simulink model "Lateral_Dynamics_2Track"  (R2020a)
settings: Solver=VariableStepAuto  StartTime=0.0  StopTime=10.0  RelTol=1e-3
values from neighbouring files (symbols this model uses):
  Brake_radius = 0.1    [Properties.sldd]
  Car_mass = 245.0    [Properties.sldd]
  CG_x = 0.6    [Properties.sldd]
  Effective_radius = 0.2    [Properties.sldd]
  Track_width = 2.0    [Properties.sldd]
  Wheel_inertia = 0.0205    [Properties.sldd]
  Wheelbase = 1.2    [Properties.sldd]
undefined symbols (not defined in the file or in its folder): Car_Iz
libraries: simulink x2
settings Model: Creator=Matthew  LastModifiedBy=Matthew

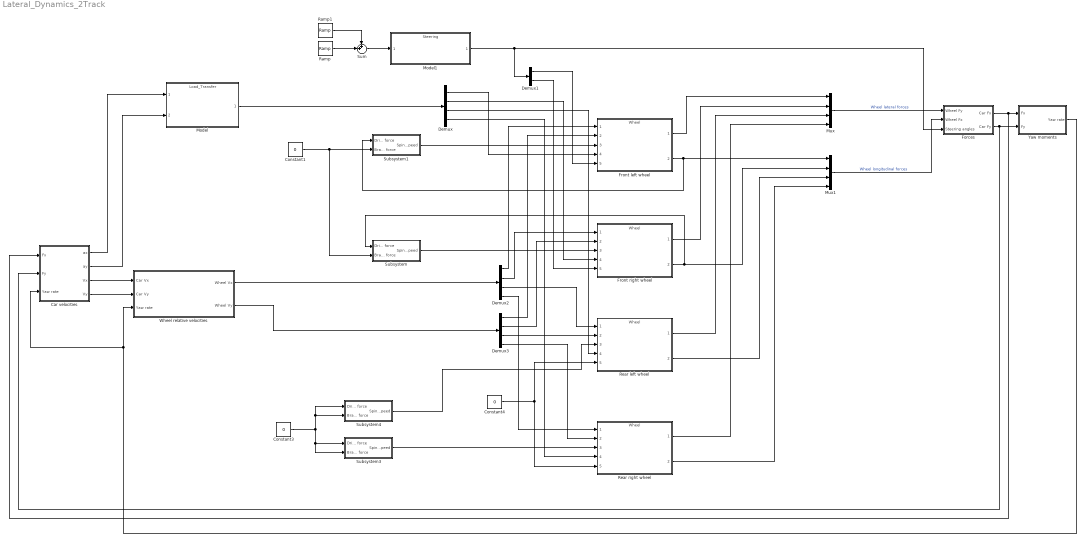
== system Lateral_Dynamics_2Track ==
  Car velocities : Subsystem
  Constant1 : Constant  Value=0
  Constant3 : Constant  Value=0
  Constant4 : Constant  Value=0
  Demux : Demux
  Demux1 : Demux  Outputs=2
  Demux2 : Demux
  Demux3 : Demux
  Forces : Subsystem
  Front left wheel : ModelReference  ModelNameDialog=Wheel  SimulationMode=Normal  ModelReferenceVersion=1.8
  Front right wheel : ModelReference  ModelNameDialog=Wheel  SimulationMode=Normal  ModelReferenceVersion=1.8
  Model : ModelReference  ModelNameDialog=Load_Transfer  SimulationMode=Normal  ModelReferenceVersion=1.23
  Model1 : ModelReference  ModelNameDialog=Steering  SimulationMode=Normal  ModelReferenceVersion=1.2
  Mux : Mux
  Mux1 : Mux
  Ramp : simulink/Sources/Ramp  slope=0.05  start=0  InitialOutput=0
  Ramp1 : simulink/Sources/Ramp  slope=-0.05  start=2  InitialOutput=0
  Rear left wheel : ModelReference  ModelNameDialog=Wheel  SimulationMode=Normal  ModelReferenceVersion=1.8
  Rear right wheel : ModelReference  ModelNameDialog=Wheel  SimulationMode=Normal  ModelReferenceVersion=1.8
  Subsystem : Subsystem
  Subsystem1 : Subsystem
  Subsystem3 : Subsystem
  Subsystem4 : Subsystem
  Sum : Sum  Inputs=++|
  Wheel relative velocities : Subsystem
  Yaw moments : Subsystem
  wires:
  Subsystem/1(Spin speed) -> Front right wheel/3
  Demux/2 -> Front right wheel/4
  Model/1 -> Demux/1
  Subsystem1/1(Spin speed) -> Front left wheel/3
  Car velocities/1(ax) -> Model/1
  Demux/1 -> Front left wheel/4
  Front left wheel/1 -> Mux/1
  Front right wheel/1 -> Mux/2
  Constant1/1 -> Subsystem/2(Brake force), Subsystem1/2(Brake force)
  Wheel relative velocities/1(Wheel Vx) -> Demux2/1
  Wheel relative velocities/2(Wheel Vy) -> Demux3/1
  Demux2/1 -> Front left wheel/1
  Demux3/1 -> Front left wheel/2
  Demux2/2 -> Front right wheel/1
  Demux3/2 -> Front right wheel/2
  Subsystem4/1(Spin speed) -> Rear left wheel/3
  Constant3/1 -> Subsystem4/2(Brake force), Subsystem4/1(Drive force), Subsystem3/2(Brake force), Subsystem3/1(Drive force)
  Rear left wheel/1 -> Mux/3
  Rear right wheel/1 -> Mux/4
  Front left wheel/2 -> Subsystem1/1(Drive force), Mux1/1
  Front right wheel/2 -> Subsystem/1(Drive force), Mux1/2
  Rear left wheel/2 -> Mux1/3
  Rear right wheel/2 -> Mux1/4
  Mux/1 -> Forces/1(Wheel Fy)  "Wheel lateral forces"
  Mux1/1 -> Forces/2(Wheel Fx)  "Wheel longitudinal forces"
  Model1/1 -> Forces/3(Steering angles), Demux1/1
  Constant4/1 -> Rear left wheel/5, Rear right wheel/5
  Subsystem3/1(Spin speed) -> Rear right wheel/3
  Demux2/3 -> Rear left wheel/1
  Demux2/4 -> Rear right wheel/1
  Demux3/3 -> Rear left wheel/2
  Demux3/4 -> Rear right wheel/2
  Demux1/1 -> Front left wheel/5
  Demux1/2 -> Front right wheel/5
  Forces/1(Car Fx) -> Car velocities/1(Fx), Yaw moments/1(Fx)
  Forces/2(Car Fy) -> Car velocities/2(Fy), Yaw moments/2(Fy)
  Yaw moments/1(Yaw rate) -> Car velocities/3(Yaw rate), Wheel relative velocities/3(Yaw rate)
  Demux/3 -> Rear left wheel/4
  Demux/4 -> Rear right wheel/4
  Car velocities/3(Vx) -> Wheel relative velocities/1(Car Vx)
  Car velocities/4(Vy) -> Wheel relative velocities/2(Car Vy)
  Car velocities/2(ay) -> Model/2
  Sum/1 -> Model1/1
  Ramp1/1 -> Sum/1
  Ramp/1 -> Sum/2

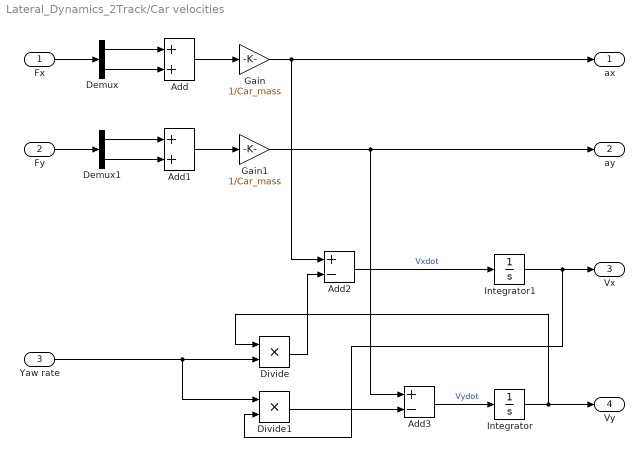
== system Lateral_Dynamics_2Track/Car velocities ==
  Fx : Inport
  Fy : Inport  Port=2
  Yaw rate : Inport  Port=3
  Add : Sum  Inputs=2
  Add1 : Sum  Inputs=2
  Add2 : Sum  Inputs=+-
  Add3 : Sum  Inputs=+-
  Demux : Demux  Outputs=2
  Demux1 : Demux  Outputs=2
  Divide : Product  Inputs=**
  Divide1 : Product  Inputs=**
  Gain : Gain  Gain=1/Car_mass
  Gain1 : Gain  Gain=1/Car_mass
  Integrator : Integrator
  Integrator1 : Integrator
  ax : Outport
  ay : Outport  Port=2
  Vx : Outport  Port=3
  Vy : Outport  Port=4
  wires:
  Fx/1 -> Demux/1
  Demux/1 -> Add/1
  Demux/2 -> Add/2
  Fy/1 -> Demux1/1
  Demux1/1 -> Add1/1
  Demux1/2 -> Add1/2
  Add/1 -> Gain/1
  Add1/1 -> Gain1/1
  Gain/1 -> ax/1, Add2/1
  Gain1/1 -> Add3/1, ay/1
  Integrator1/1 -> Divide1/2, Vx/1
  Integrator/1 -> Vy/1, Divide/1
  Yaw rate/1 -> Divide1/1, Divide/2
  Divide/1 -> Add2/2
  Divide1/1 -> Add3/2
  Add3/1 -> Integrator/1  "Vydot"
  Add2/1 -> Integrator1/1  "Vxdot"

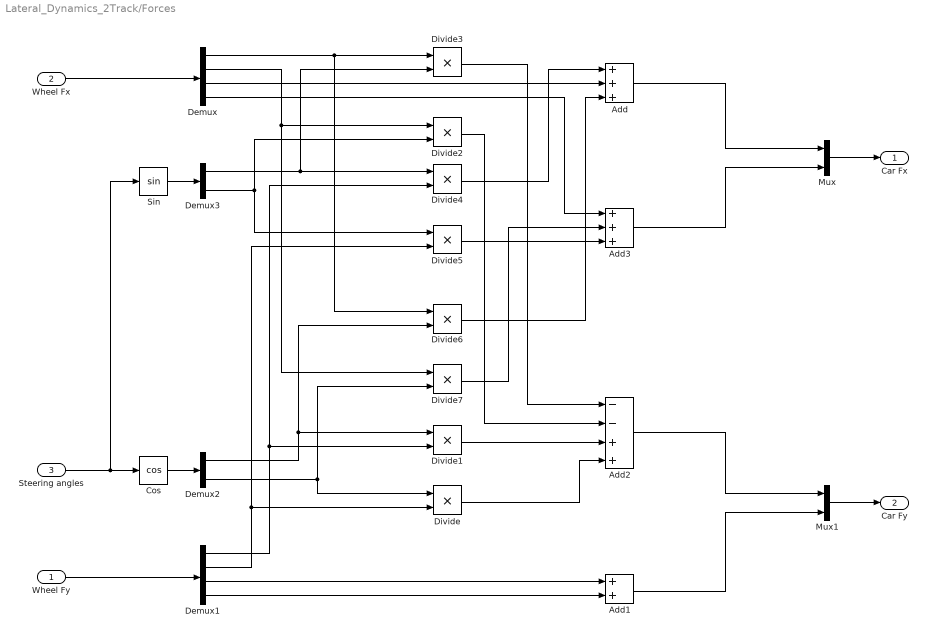
== system Lateral_Dynamics_2Track/Forces ==
  Wheel Fy : Inport
  Wheel Fx : Inport  Port=2
  Steering angles : Inport  Port=3
  Add : Sum  Inputs=3
  Add1 : Sum  Inputs=2
  Add2 : Sum  Inputs=--++
  Add3 : Sum  Inputs=3
  Cos : Trigonometry  Operator=cos
  Demux : Demux
  Demux1 : Demux
  Demux2 : Demux  Outputs=2
  Demux3 : Demux  Outputs=2
  Divide{,1..3,6..7} (6 alike) : Product  Inputs=**
  Divide4 : Product
  Divide5 : Product
  Mux : Mux  Inputs=2
  Mux1 : Mux  Inputs=2
  Sin : Trigonometry
  Car Fx : Outport
  Car Fy : Outport  Port=2
  wires:
  Wheel Fx/1 -> Demux/1
  Wheel Fy/1 -> Demux1/1
  Steering angles/1 -> Sin/1, Cos/1
  Cos/1 -> Demux2/1
  Demux2/2 -> Divide7/2, Divide/1
  Demux1/1 -> Divide1/2, Divide4/2
  Demux1/2 -> Divide5/2, Divide/2
  Demux2/1 -> Divide6/2, Divide1/1
  Sin/1 -> Demux3/1
  Demux3/1 -> Divide4/1, Divide3/2
  Demux/1 -> Divide6/1, Divide3/1
  Demux/2 -> Divide7/1, Divide2/1
  Demux3/2 -> Divide5/1, Divide2/2
  Demux/3 -> Add/2
  Demux1/3 -> Add1/1
  Demux1/4 -> Add1/2
  Add1/1 -> Mux1/2
  Add2/1 -> Mux1/1
  Add/1 -> Mux/1
  Add3/1 -> Mux/2
  Mux/1 -> Car Fx/1
  Mux1/1 -> Car Fy/1
  Demux/4 -> Add3/1
  Divide3/1 -> Add2/1
  Divide6/1 -> Add/3
  Divide5/1 -> Add3/3
  Divide4/1 -> Add/1
  Divide2/1 -> Add2/2
  Divide7/1 -> Add3/2
  Divide1/1 -> Add2/3
  Divide/1 -> Add2/4

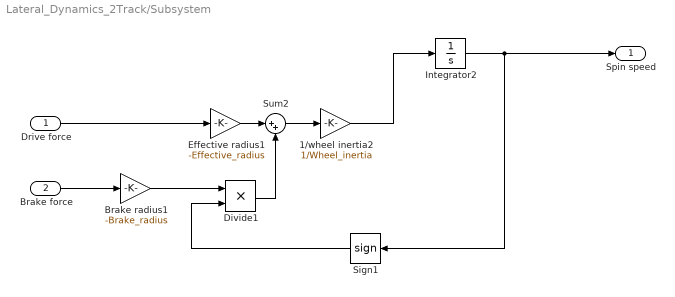
== system Lateral_Dynamics_2Track/Subsystem ==
  Drive force : Inport
  Brake force : Inport  Port=2
  1/wheel inertia2 : Gain  Gain=1/Wheel_inertia
  Brake radius1 : Gain  Gain=-Brake_radius
  Divide1 : Product  Inputs=**
  Effective radius1 : Gain  Gain=-Effective_radius
  Integrator2 : Integrator  InitialCondition=45
  Sign1 : Signum
  Sum2 : Sum  Inputs=|++
  Spin speed : Outport
  wires:
  Integrator2/1 -> Spin speed/1, Sign1/1
  Divide1/1 -> Sum2/2
  1/wheel inertia2/1 -> Integrator2/1
  Sign1/1 -> Divide1/2
  Sum2/1 -> 1/wheel inertia2/1
  Drive force/1 -> Effective radius1/1
  Brake radius1/1 -> Divide1/1
  Effective radius1/1 -> Sum2/1
  Brake force/1 -> Brake radius1/1

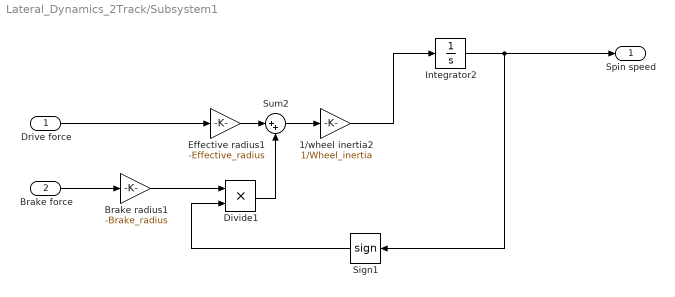
== system Lateral_Dynamics_2Track/Subsystem1 ==
  Drive force : Inport
  Brake force : Inport  Port=2
  1/wheel inertia2 : Gain  Gain=1/Wheel_inertia
  Brake radius1 : Gain  Gain=-Brake_radius
  Divide1 : Product  Inputs=**
  Effective radius1 : Gain  Gain=-Effective_radius
  Integrator2 : Integrator  InitialCondition=45
  Sign1 : Signum
  Sum2 : Sum  Inputs=|++
  Spin speed : Outport
  wires:
  Integrator2/1 -> Spin speed/1, Sign1/1
  Divide1/1 -> Sum2/2
  1/wheel inertia2/1 -> Integrator2/1
  Sign1/1 -> Divide1/2
  Sum2/1 -> 1/wheel inertia2/1
  Drive force/1 -> Effective radius1/1
  Brake radius1/1 -> Divide1/1
  Effective radius1/1 -> Sum2/1
  Brake force/1 -> Brake radius1/1

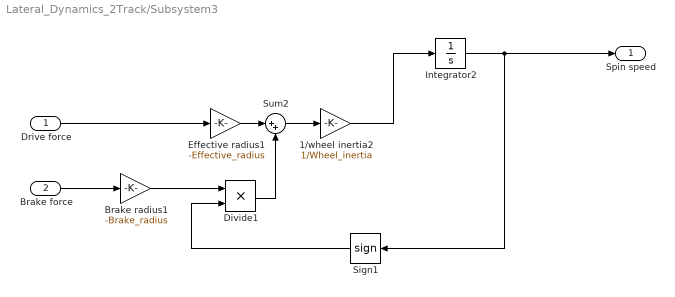
== system Lateral_Dynamics_2Track/Subsystem3 ==
  Drive force : Inport
  Brake force : Inport  Port=2
  1/wheel inertia2 : Gain  Gain=1/Wheel_inertia
  Brake radius1 : Gain  Gain=-Brake_radius
  Divide1 : Product  Inputs=**
  Effective radius1 : Gain  Gain=-Effective_radius
  Integrator2 : Integrator  InitialCondition=45
  Sign1 : Signum
  Sum2 : Sum  Inputs=|++
  Spin speed : Outport
  wires:
  Integrator2/1 -> Spin speed/1, Sign1/1
  Divide1/1 -> Sum2/2
  1/wheel inertia2/1 -> Integrator2/1
  Sign1/1 -> Divide1/2
  Sum2/1 -> 1/wheel inertia2/1
  Drive force/1 -> Effective radius1/1
  Brake radius1/1 -> Divide1/1
  Effective radius1/1 -> Sum2/1
  Brake force/1 -> Brake radius1/1

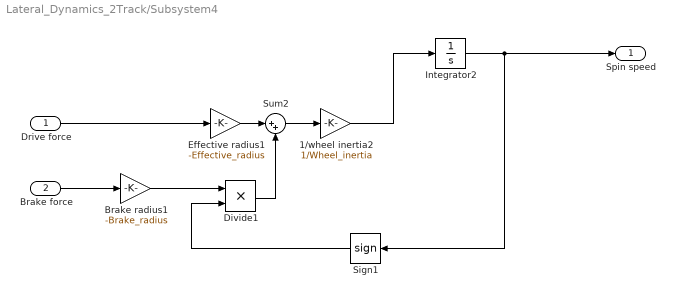
== system Lateral_Dynamics_2Track/Subsystem4 ==
  Drive force : Inport
  Brake force : Inport  Port=2
  1/wheel inertia2 : Gain  Gain=1/Wheel_inertia
  Brake radius1 : Gain  Gain=-Brake_radius
  Divide1 : Product  Inputs=**
  Effective radius1 : Gain  Gain=-Effective_radius
  Integrator2 : Integrator  InitialCondition=45
  Sign1 : Signum
  Sum2 : Sum  Inputs=|++
  Spin speed : Outport
  wires:
  Integrator2/1 -> Spin speed/1, Sign1/1
  Divide1/1 -> Sum2/2
  1/wheel inertia2/1 -> Integrator2/1
  Sign1/1 -> Divide1/2
  Sum2/1 -> 1/wheel inertia2/1
  Drive force/1 -> Effective radius1/1
  Brake radius1/1 -> Divide1/1
  Effective radius1/1 -> Sum2/1
  Brake force/1 -> Brake radius1/1

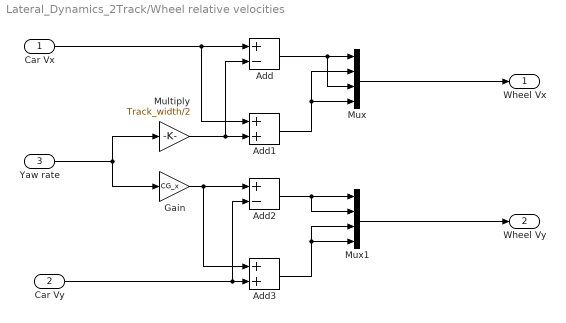
== system Lateral_Dynamics_2Track/Wheel relative velocities ==
  Car Vx : Inport
  Car Vy : Inport  Port=2
  Yaw rate : Inport  Port=3
  Add : Sum  Inputs=+-
  Add1 : Sum  Inputs=2
  Add2 : Sum  Inputs=+-
  Add3 : Sum  Inputs=2
  Gain : Gain  Gain=CG_x
  Multiply : Gain  Gain=Track_width/2
  Mux : Mux
  Mux1 : Mux
  Wheel Vx : Outport
  Wheel Vy : Outport  Port=2
  wires:
  Yaw rate/1 -> Multiply/1, Gain/1
  Car Vx/1 -> Add1/1, Add/1
  Multiply/1 -> Add1/2, Add/2
  Add/1 -> Mux/3, Mux/1
  Add1/1 -> Mux/4, Mux/2
  Mux/1 -> Wheel Vx/1
  Add3/1 -> Mux1/3, Mux1/4
  Gain/1 -> Add2/1, Add3/1
  Car Vy/1 -> Add2/2, Add3/2
  Add2/1 -> Mux1/2, Mux1/1
  Mux1/1 -> Wheel Vy/1

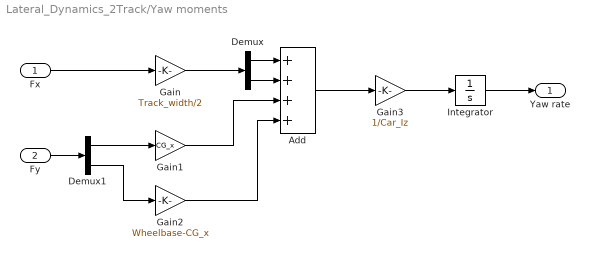
== system Lateral_Dynamics_2Track/Yaw moments ==
  Fx : Inport
  Fy : Inport  Port=2
  Add : Sum  Inputs=4
  Demux : Demux  Outputs=2
  Demux1 : Demux  Outputs=2
  Gain : Gain  Gain=Track_width/2
  Gain1 : Gain  Gain=CG_x
  Gain2 : Gain  Gain=Wheelbase-CG_x
  Gain3 : Gain  Gain=1/Car_Iz
  Integrator : Integrator
  Yaw rate : Outport
  wires:
  Integrator/1 -> Yaw rate/1
  Fx/1 -> Gain/1
  Add/1 -> Gain3/1
  Gain/1 -> Demux/1
  Demux/1 -> Add/1
  Demux/2 -> Add/2
  Gain1/1 -> Add/3
  Fy/1 -> Demux1/1
  Demux1/1 -> Gain1/1
  Demux1/2 -> Gain2/1
  Gain2/1 -> Add/4
  Gain3/1 -> Integrator/1
